simulink model "Digital_LeadLag_System_Ramp"  (R2024a)
settings: Solver=VariableStepAuto  StartTime=0.0  StopTime=10.0  RelTol=1e-3
libraries: simulink x1
settings Model: Creator=parthivkukadia  LastModifiedBy=parthivkukadia

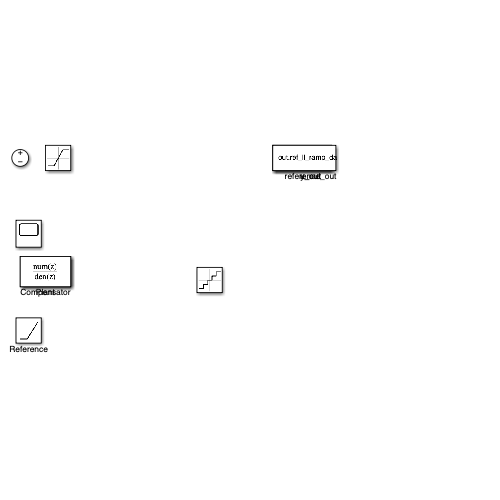
[thumbnail: Simulink's stored preview of the top-level diagram]
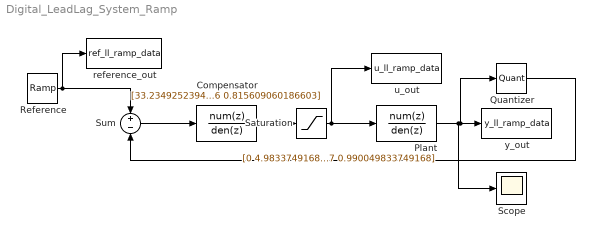
== system Digital_LeadLag_System_Ramp ==
  Compensator : DiscreteTransferFcn  Numerator=[33.2349252394128 -65.9638838359153 32.7291747414072]  Denominator=[1 -1.81560581518726 0.815609060186603]  SampleTime=0.01
  Plant : DiscreteTransferFcn  Numerator=[0 4.98337491680535e-05 4.9667913340266e-05]  Denominator=[1 -1.99004983374917 0.990049833749168]  SampleTime=0.01
  Quantizer : Quantizer  QuantizationInterval=0.0062832
  Reference : simulink/Sources/Ramp  slope=1  start=0  InitialOutput=0
  Saturation : Saturate  UpperLimit=5  LowerLimit=-5
  Scope : Scope
  Sum : Sum  Inputs=+-
  reference_out : ToWorkspace  VariableName=ref_ll_ramp_data  SaveFormat=Timeseries  SampleTime=-1
  u_out : ToWorkspace  VariableName=u_ll_ramp_data  SaveFormat=Timeseries  SampleTime=-1
  y_out : ToWorkspace  VariableName=y_ll_ramp_data  SaveFormat=Timeseries  SampleTime=-1
  wires:
  Quantizer/1 -> Sum/2
  Saturation/1 -> u_out/1, Plant/1
  Compensator/1 -> Saturation/1
  Reference/1 -> reference_out/1, Sum/1
  Sum/1 -> Compensator/1
  Plant/1 -> y_out/1, Quantizer/1, Scope/1
